simulink model "Sim2Twin_controlsystem_spd"  (R2024b)
settings: Solver=VariableStepAuto  StartTime=0.0  StopTime=10.0  RelTol=1e-3
settings Model: Creator=Emila  LastModifiedBy=Emila

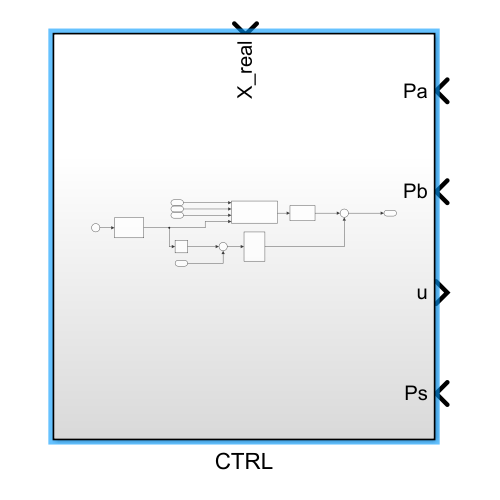
[thumbnail: Simulink's stored preview of the top-level diagram]
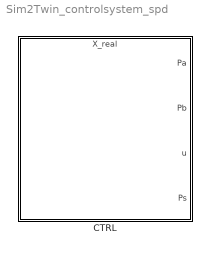
== system Sim2Twin_controlsystem_spd ==
  CTRL : Subsystem
      settings: PortSchema="{\"entries\":[{\"content\":{\"sides\":[{\"content\":{},\"type\":\"ConnectorPlacement.EquallySpacedRectSide\",\"uuid\":\"e7dc98bc-0c39-42fc-9d44-5c528a861935\"},{\"content\":{\"connectorIds\":[\"In2\",\"In3\",\"Out1\",\"In4\"],\"side\":\"RIGHT\"},\"type\":\"ConnectorPlacement.EquallySpacedRectSide\",\"uuid\":\"7a7fb2e4-7f4e-4840-80a8-3a9723ecfbf6\"},{\"content\":{\"connectorIds\":[\"In1\"],\"side\":\"TOP\"},\"type\":\"ConnectorPlacement.EquallySpacedRectSide\",\"uuid\":\"8314552e-40ce-493a-a910-ea6a3ee6c4fc\"}]},\"type\":\"ConnectorPlacement.EquallySpacedConnector\",\"uuid\":\"904788e7-187d-4514-a00a-56ca1dbc298c\"}],\"packageUris\":[\"http://schema.mathworks.com/mf0/Connector/R2020b\"],\"version\":\"1.0\"}"

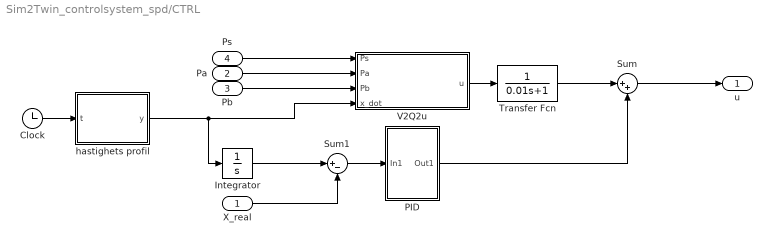
== system Sim2Twin_controlsystem_spd/CTRL ==
  X_real : Inport
  Pa : Inport  Port=2
  Pb : Inport  Port=3
  Ps : Inport  Port=4
  Clock : Clock
  Integrator : Integrator
  PID : Subsystem
  Sum : Sum  Inputs=|++
  Sum1 : Sum  Inputs=|+-
  Transfer Fcn : TransferFcn  Denominator=[0.01 1]
  V2Q2u : MATLAB Function  TreatAsAtomicUnit=on
  hastighets profil : MATLAB Function  TreatAsAtomicUnit=on
  u : Outport
  wires:
  X_real/1 -> Sum1/2
  Pb/1 -> V2Q2u/3(Pb)
  Pa/1 -> V2Q2u/2(Pa)
  Ps/1 -> V2Q2u/1(Ps)
  Clock/1 -> hastighets profil/1(t)
  hastighets profil/1(y) -> Integrator/1, V2Q2u/4(x_dot)
  Integrator/1 -> Sum1/1
  V2Q2u/1(u) -> Transfer Fcn/1
  Transfer Fcn/1 -> Sum/1
  Sum/1 -> u/1
  PID/1(Out1) -> Sum/2
  Sum1/1 -> PID/1(In1)

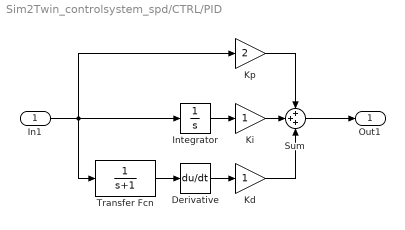
== system Sim2Twin_controlsystem_spd/CTRL/PID ==
  In1 : Inport
  Derivative : Derivative
  Integrator : Integrator
  Kd : Gain
  Ki : Gain
  Kp : Gain  Gain=2
  Sum : Sum  Inputs=+++
  Transfer Fcn : TransferFcn  Denominator=[1 1]
  Out1 : Outport
  wires:
  Integrator/1 -> Ki/1
  Derivative/1 -> Kd/1
  In1/1 -> Transfer Fcn/1, Integrator/1, Kp/1
  Sum/1 -> Out1/1
  Kd/1 -> Sum/3
  Kp/1 -> Sum/1
  Ki/1 -> Sum/2
  Transfer Fcn/1 -> Derivative/1

== matlab function Sim2Twin_controlsystem_spd/CTRL/hastighets profil ==
  data: y output; t input
function y  = fcn(t)
v_max = 0.1;
v_0 = 0;
x_0 = 0;
x_max = 0.05;
x_max = 0.25;
t_ramp = 1;
v_ref = x_max/t_ramp;
start_time = 1;
hold_time = 1;
if v_ref>v_max
    v_ref=v_max;
    y=0;
end
t1 = start_time;
t2 = t1 + t_ramp;
t3 = t2 + hold_time;
t4 = t3 + t_ramp; 
t5 = t4 + start_time;
t6 = t5 + t_ramp;
t7 = t6 + hold_time;
t8 = t7 + t_ramp;
t9 = t8 + start_time;
if t < t1
    y = x_0;
elseif t < t2 % ramp up speed
    y = x_0 + v_0*(t-t1) + v_ref*(t-t1);
elseif t < t3 %holding speed
    y = x_0 + v_ref*t_ramp;
elseif t < t4 %ramping down speed
    y = x_0 + v_ref*t_ramp - v_ref*(t-t3);
elseif t < t5 %holding 0
    y = x_0;

elseif t < t6 %ramping down speed
    y = x_0 - v_0*(t-t5) - v_ref*(t-t5);
elseif t < t7 %holdin speed
    y = x_0 - v_ref*t_ramp;
elseif t < t8 %ramping up speed
    y = x_0 - v_ref*t_ramp + v_ref*(t-t7);
elseif t < t9 %holding 0
    y = x_0;
end

== matlab function Sim2Twin_controlsystem_spd/CTRL/V2Q2u ==
  data: Ps input; Pa input; Pb input; x_dot input; u output
function u = fcn(Ps, Pa, Pb, x_dot)

phi = 0.7130;
A = 33.1/100^2; % Area
BW = 0; % deadband
SpoolTravel = 7; % Maximum Spool Travel
a = (SpoolTravel-BW)/25; % Valve Slope Characteristic [mm/(L/min)]
dP_0 = 7e5; % Pressure drop with compansator

if x_dot > 0
    Q = x_dot * A; % Wanted Flow
    dP = (Ps-Pa)*1e5;
    dp_ref = abs(dP_0/dP);
    %dp_ref = 1;
    Q_star = (Q * sqrt(dp_ref)) * 6e4; % Referance Flow [L/min]
    u = (Q_star * a + BW)/SpoolTravel; % Control Signal [-1, 1]

elseif x_dot < 0
    Q = x_dot * (A*phi); % Wanted Flow
    dP = (Ps-Pb)*1e5;
    dp_ref = abs(dP_0/dP);
   % dp_ref = 1;
    Q_star = (Q * sqrt(dp_ref)) * 6e4; % Referance Flow [L/min]
    u = (Q_star * a - BW)/SpoolTravel; % Control Signal [-1, 1]

else
    u = 0;

end
end
